simulink model "pv2grid_boost_inverter_mppt_irradiation"  (R2019a)
settings: Solver=FixedStepDiscrete  StartTime=0.0  StopTime=4  FixedStep=Ts  RelTol=1e-3
values from neighbouring files (symbols this model uses):
  Ts = 1e-05    [variablTable.mat]
undefined symbols (not defined in the file or in its folder): sigbuilder_block
libraries: powerlib x1
settings Model: Creator=ng  LastModifiedBy=ng

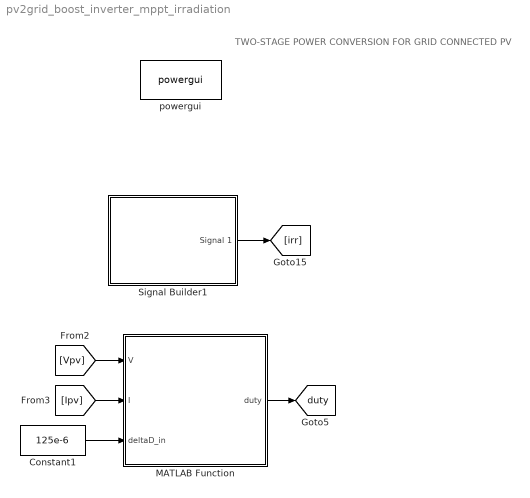
== system pv2grid_boost_inverter_mppt_irradiation ==
  note: TWO-STAGE POWER CONVERSION FOR
      | GRID CONNECTED PV
  Constant1 : Constant  Value=125e-6
  MATLAB Function : MATLAB Function  TreatAsAtomicUnit=on
  Signal Builder1 : Subsystem  Tag=STV Subsys  LoadFcn=sigbuilder_block('load');  StartFcn=sigbuilder_block('start');  StopFcn=sigbuilder_block('stop');  ClipboardFcn=sigbuilder_block('clipboard');  mask(Sigbuilder block){tuvar=[0:10]}
      mask help: Simulink:masks:SigbuilderBlock_MD
      mask init:
      | if ~strcmp(get_param(bdroot(gcbh),'SimulationStatus'),'stopped') tuvar = sigbuilder_block('maskInit'); end
      settings: CopyFcn=sigbuilder_block('copy');  DeleteFcn=sigbuilder_block('delete');  ModelCloseFcn=sigbuilder_block('modelClose');  PreSaveFcn=sigbuilder_block('preSave');  PauseFcn=sigbuilder_block('pause');  ContinueFcn=sigbuilder_block('continue');  NameChangeFcn=sigbuilder_block('namechange');  OpenFcn=sigbuilder_block('open',[220.2 153.6 550.8 361.2 ]);  CloseFcn=sigbuilder_block('close');
      mask Display: plot(0, 0, 100, 100,[2, 2, 32, 32, 2], [68, 8, 8, 68, 68],[32, 2], [38, 38], [32, 19, 2],[53, 60, 44], [32, 17, 17, 2],[16, 16, 31, 31]);txt = getActiveGroup(gcbh);text(2, 100, txt,'verticalAlignment', 'top');
  powergui : powerlib/powergui  Priority=1  SimulationMode=Discrete  SampleTime=Ts  frequency=60  Iterations=50  frequencyindice=0  Pbase=100e6  ErrMax=1e-4  UnitsV=kV  UnitsW=MW  buscounter=0  FunctionMessages=off  echomessages=off  EnableUseOfTLC=off  CurrentSourceSwitches=off  DisableSnubberDevices=off  DisableRonSwitches=off  DisableVfSwitches=off  DisplayEquations=off  AutomaticDiscreteSolvers=off  SolverType=Tustin/Backward Euler (TBE)  Interpol=off  ExternalGateDelay=off  methode=off  Ts=100  x0status=blocks  SPID=on  SwTol=0  HookPort=off  NonlinearTolerance=0  nMaxIteration=15  ContinueOnMaxIteration=off  RestoreLinks=warning  ResistiveCurrentMeasurement=off  Frange=[0:2:500]  Ylog=off  Xlog=on  ShowGrid=off  save=off  variable=ZData  structure=0  ZoomFFT=off  StartTime=0.0  cycles=1  DisplayStyle=1  fundamental=60  FreqAxis=off  MaxFrequency=1000  frequencyindicesteady=1  RmsSteady=1  display=off
      settings: SourceProductName=Simscape Electrical
  tag scope: duty=global
  wires:
  Signal Builder1/1(Signal 1) -> [irr]
  [Vpv] -> MATLAB Function/1(V)
  [Ipv] -> MATLAB Function/2(I)
  Constant1/1 -> MATLAB Function/3(deltaD_in)
  MATLAB Function/1(duty) -> [duty]

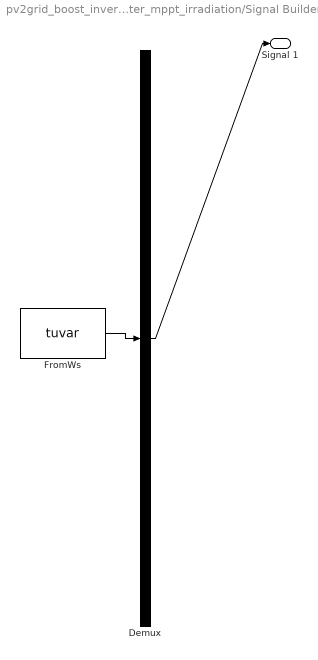
== system pv2grid_boost_inverter_mppt_irradiation/Signal Builder1 ==
  Demux : Demux  Tag=STV Demux  Outputs=1
  FromWs : FromWorkspace  Tag=STV FromWs  VariableName=tuvar  SampleTime=0
      SigBuilderData=|
      | common.afterFinalStr = 'Extrapolate'
      | common.sampleTime = 0
      | dataSet.timeRange = [0 4]
      | dataSet.name = 'Group 1'
      | sbobj.Groups.Name = 'Group 1'
      | sbobj.Groups.Signals.Name = 'Signal 1'
      | sbobj.Groups.Signals.XData = [0 0.00416233090531 0.00832466181061 0.0124869927159 0.0166493236212 0.0208116545265 0.0249739854318 0.0291363163371 0.0332986472425 0.0374609781478 0.0416233090531 0.0457856399584 ... (962 elements, 1x962)]
      | sbobj.Groups.Signals.YData = [2.47122187864 2.47122187864 2.47122187864 2.47122187864 2.47122187864 2.47122187864 2.47122187864 2.47122187864 2.47122187864 2.47121149505 2.47121149505 2.47121149505 ... (962 elements, 1x962)]
      | sbobj.Groups.TimeRange = [0 4]
  Signal 1 : Outport  Tag=STV Outport
  wires:
  FromWs/1 -> Demux/1
  Demux/1 -> Signal 1/1

== matlab function pv2grid_boost_inverter_mppt_irradiation/MATLAB Function ==
  data: V input; duty output; I input; deltaD_in input
function duty = MPPT_Kontrol( V, I,deltaD_in)

duty_init = 0.05;
duty_min=0;
duty_max=0.75;

persistent Vold Pold duty_old;

if isempty(Vold)
    Vold=0;
    Pold=0;
    duty_old=duty_init;
end
P= V*I;
dV= V - Vold;
dP= P - Pold;
duty = duty_old;
deltaD=deltaD_in;

if dP ~= 0
    if dP < 0
        if dV < 0
            duty = duty_old - deltaD;
        else
            duty = duty_old + deltaD;
        end
    else
        if dV < 0
            duty = duty_old + deltaD;
        else
            duty = duty_old - deltaD;
        end
    end
end

if duty >= duty_max
    duty=duty_max;
elseif duty<duty_min
    duty=duty_min;
end

duty_old=duty;
Vold=V;
Pold=P;
